simulink model "Single_FLL"  (R2021a)
settings: Solver=VariableStepAuto  StartTime=0.0  StopTime=2  RelTol=1e-3
libraries: dspswit3 x2, spspowerguiLib x1
settings Model: Creator=Swaran Pratap Singh  LastModifiedBy=Swaran Pratap Singh
settings DataIOCC: InspectSignalLogs=on  ReturnWorkspaceOutputs=off

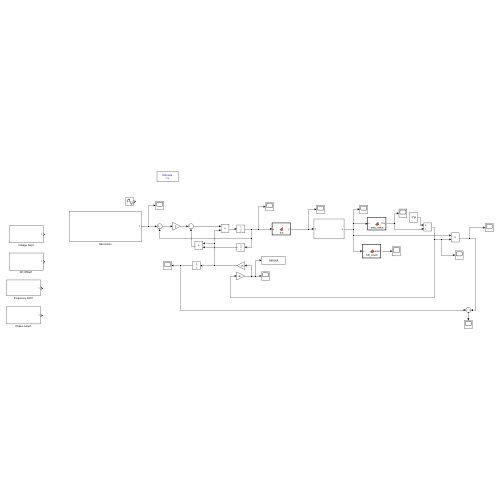
[thumbnail: Simulink's stored preview of the top-level diagram]
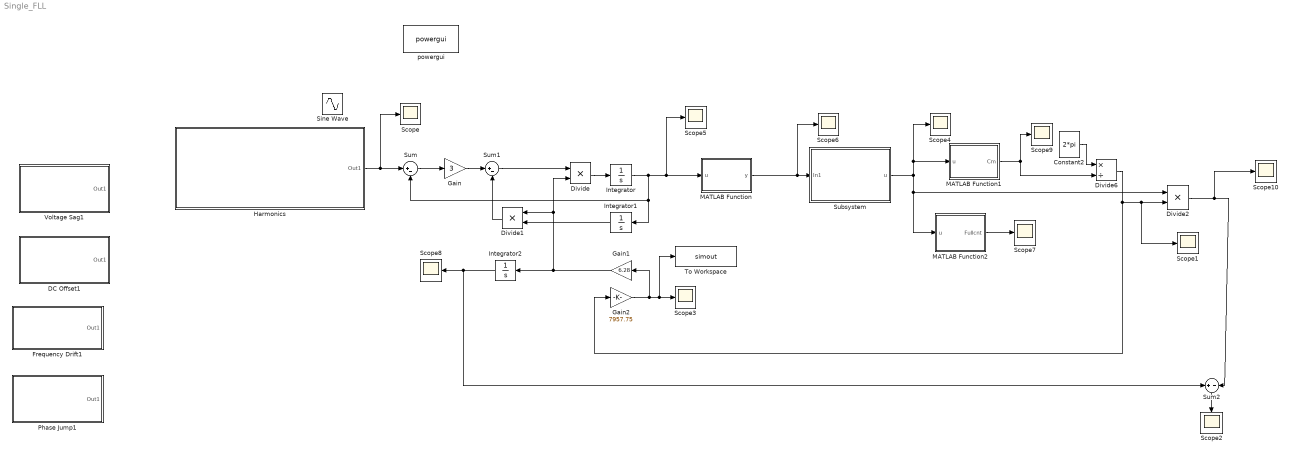
== system Single_FLL ==
  Constant2 : Constant  Value=2*pi
  DC Offset1 : Subsystem
  Divide : Product  Inputs=**
  Divide1 : Product  Inputs=**
  Divide2 : Product  Inputs=**
  Divide6 : Product  Inputs=*/
  Frequency Drift1 : Subsystem
  Gain : Gain  Gain=3
  Gain1 : Gain  Gain=6.28
  Gain2 : Gain  Gain=7957.75
  Harmonics : Subsystem
  Integrator : Integrator
  Integrator1 : Integrator
  Integrator2 : Integrator
  MATLAB Function : MATLAB Function  TreatAsAtomicUnit=on
  MATLAB Function1 : MATLAB Function  TreatAsAtomicUnit=on
  MATLAB Function2 : MATLAB Function  TreatAsAtomicUnit=on
  Phase Jump1 : Subsystem
  Scope{,1..10} (11 alike) : Scope
  Sine Wave : Sin  Amplitude=230  Frequency=2*pi*50  SampleTime=0.000001
  Subsystem : Subsystem
  Sum : Sum  Inputs=|+-
  Sum1 : Sum  Inputs=|+-
  Sum2 : Sum  Inputs=+-
  To Workspace : ToWorkspace  VariableName=simout  SaveFormat=Timeseries  SampleTime=-1
  Voltage Sag1 : Subsystem
  powergui : spspowerguiLib/powergui  Priority=1  SimulationMode=Discrete  SampleTime=1  frequency=60  Iterations=50  frequencyindice=50  Pbase=100e6  ErrMax=1e-4  UnitsV=kV  UnitsW=MW  buscounter=0  FunctionMessages=off  echomessages=off  EnableUseOfTLC=off  CurrentSourceSwitches=off  DisableSnubberDevices=off  DisableRonSwitches=off  DisableVfSwitches=off  DisplayEquations=off  AutomaticDiscreteSolvers=off  SolverType=Tustin/Backward Euler (TBE)  Interpol=off  ExternalGateDelay=off  methode=off  Ts=100  x0status=blocks  SPID=on  SwTol=0  HookPort=off  NonlinearTolerance=1e-4  nMaxIteration=100  ContinueOnMaxIteration=off  RestoreLinks=warning  ResistiveCurrentMeasurement=off  Frange=[0:2:500]  Ylog=off  Xlog=on  ShowGrid=off  save=off  variable=ZData  structure=0  ZoomFFT=off  StartTime=0.0  cycles=1  DisplayStyle=1  fundamental=60  FreqAxis=off  MaxFrequency=1000  frequencyindicesteady=1  RmsSteady=1  display=off
  wires:
  MATLAB Function/1(y) -> Scope6/1, Subsystem/1(In1)
  Subsystem/1(u) -> MATLAB Function1/1(u), Scope4/1, MATLAB Function2/1(u), Divide2/1
  Gain1/1 -> Integrator2/1, Divide1/1, Divide/2
  Sum/1 -> Gain/1
  Divide2/1 -> Scope10/1, Sum2/2
  Integrator1/1 -> Divide1/2
  Divide1/1 -> Sum1/2
  Gain/1 -> Sum1/1
  Constant2/1 -> Divide6/1
  MATLAB Function2/1(Fullcnt) -> Scope7/1
  Divide/1 -> Integrator/1
  Integrator2/1 -> Sum2/1, Scope8/1
  MATLAB Function1/1(Cm) -> Divide6/2, Scope9/1
  Gain2/1 -> To Workspace/1, Scope3/1, Gain1/1
  Sum2/1 -> Scope2/1
  Divide6/1 -> Gain2/1, Scope1/1, Divide2/2
  Sum1/1 -> Divide/1
  Integrator/1 -> Integrator1/1, Sum/2, Scope5/1, MATLAB Function/1(u)
  Harmonics/1(Out1) -> Scope/1, Sum/1

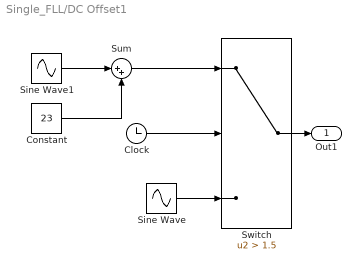
== system Single_FLL/DC Offset1 ==
  Clock : Clock
  Constant : Constant  Value=23
  Sine Wave : Sin  Amplitude=230  Frequency=314.16  SampleTime=0.000001
  Sine Wave1 : Sin  Amplitude=230  Frequency=314.16  SampleTime=0.000001
  Sum : Sum  Inputs=|++
  Switch : Switch  Criteria=u2 > Threshold  Threshold=1.5
  Out1 : Outport
  wires:
  Clock/1 -> Switch/2
  Sine Wave/1 -> Switch/3
  Switch/1 -> Out1/1
  Sine Wave1/1 -> Sum/1
  Constant/1 -> Sum/2
  Sum/1 -> Switch/1

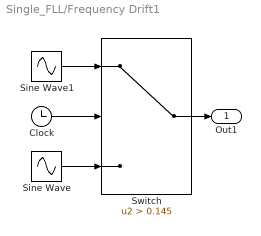
== system Single_FLL/Frequency Drift1 ==
  Clock : Clock
  Sine Wave : Sin  Amplitude=230  Frequency=314.16  SampleTime=0.000001
  Sine Wave1 : Sin  Amplitude=230  Frequency=333.01  Phase=pi  SampleTime=0.000001
  Switch : Switch  Criteria=u2 > Threshold  Threshold=0.145
  Out1 : Outport
  wires:
  Sine Wave1/1 -> Switch/1
  Sine Wave/1 -> Switch/3
  Clock/1 -> Switch/2
  Switch/1 -> Out1/1

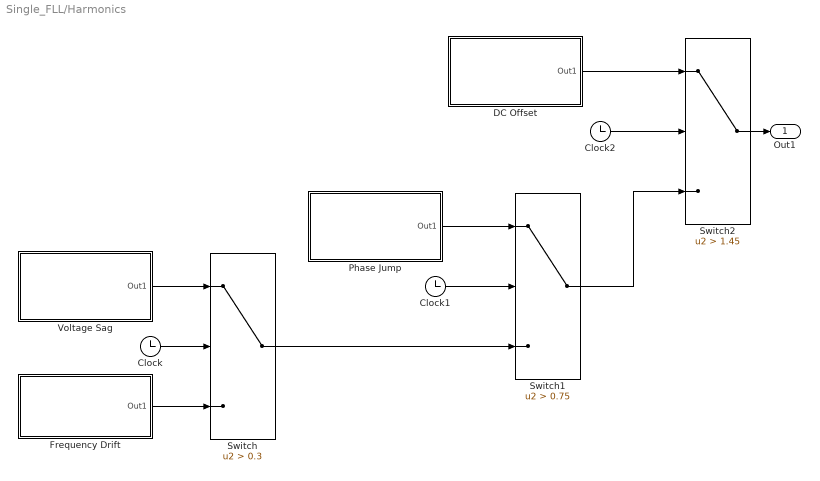
== system Single_FLL/Harmonics ==
  Clock : Clock
  Clock1 : Clock
  Clock2 : Clock
  DC Offset : Subsystem
  Frequency Drift : Subsystem
  Phase Jump : Subsystem
  Switch : Switch  Criteria=u2 > Threshold  Threshold=0.3
  Switch1 : Switch  Criteria=u2 > Threshold  Threshold=0.75
  Switch2 : Switch  Criteria=u2 > Threshold  Threshold=1.45
  Voltage Sag : Subsystem
  Out1 : Outport
  wires:
  Phase Jump/1(Out1) -> Switch1/1
  Switch1/1 -> Switch2/3
  DC Offset/1(Out1) -> Switch2/1
  Switch/1 -> Switch1/3
  Clock/1 -> Switch/2
  Clock1/1 -> Switch1/2
  Frequency Drift/1(Out1) -> Switch/3
  Clock2/1 -> Switch2/2
  Voltage Sag/1(Out1) -> Switch/1
  Switch2/1 -> Out1/1

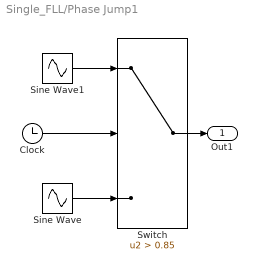
== system Single_FLL/Phase Jump1 ==
  Clock : Clock
  Sine Wave : Sin  Amplitude=230  Frequency=314.16  SampleTime=0.000001
  Sine Wave1 : Sin  Amplitude=230  Frequency=314.16  Phase=0.4167*pi  SampleTime=0.000001
  Switch : Switch  Criteria=u2 > Threshold  Threshold=0.85
  Out1 : Outport
  wires:
  Clock/1 -> Switch/2
  Sine Wave1/1 -> Switch/1
  Sine Wave/1 -> Switch/3
  Switch/1 -> Out1/1

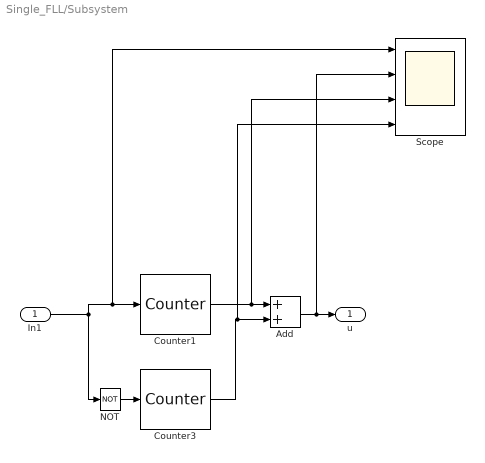
== system Single_FLL/Subsystem ==
  In1 : Inport
  Add : Sum
  Counter1 : dspswit3/Counter  Direction=Up  CountEvent=Free running  CounterSize=User defined  MaxCount=10000  InitialCount=0  Output=Count  HitValue=32  ResetInput=on  SamplesPerFrame=1  Ts=0.00001  CntDtype=double  HitDtype=Logical
  Counter3 : dspswit3/Counter  Direction=Up  CountEvent=Free running  CounterSize=User defined  MaxCount=10000  InitialCount=0  Output=Count  HitValue=32  ResetInput=on  SamplesPerFrame=1  Ts=0.00001  CntDtype=double  HitDtype=Logical
  NOT : Logic  Operator=NOT  IconShape=distinctive  AllPortsSameDT=off  OutDataTypeStr=boolean
  Scope : Scope  NumInputPorts=4
  u : Outport
  wires:
  NOT/1 -> Counter3/1
  Counter3/1 -> Scope/4, Add/2
  Counter1/1 -> Scope/3, Add/1
  In1/1 -> NOT/1, Scope/1, Counter1/1
  Add/1 -> Scope/2, u/1

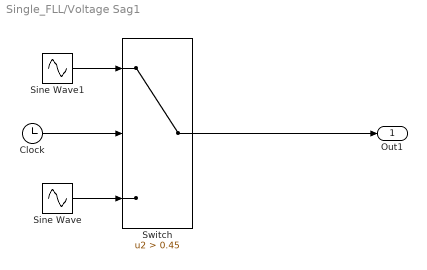
== system Single_FLL/Voltage Sag1 ==
  Clock : Clock
  Sine Wave : Sin  Amplitude=230  Frequency=314.16  SampleTime=0.000001
  Sine Wave1 : Sin  Amplitude=138  Frequency=314.16  SampleTime=0.000001
  Switch : Switch  Criteria=u2 > Threshold  Threshold=0.45
  Out1 : Outport
  wires:
  Clock/1 -> Switch/2
  Sine Wave1/1 -> Switch/1
  Sine Wave/1 -> Switch/3
  Switch/1 -> Out1/1

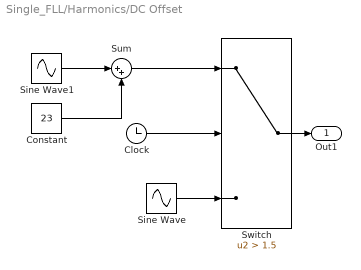
== system Single_FLL/Harmonics/DC Offset ==
  Clock : Clock
  Constant : Constant  Value=23
  Sine Wave : Sin  Amplitude=230  Frequency=314.16  SampleTime=0.000001
  Sine Wave1 : Sin  Amplitude=230  Frequency=314.16  SampleTime=0.000001
  Sum : Sum  Inputs=|++
  Switch : Switch  Criteria=u2 > Threshold  Threshold=1.5
  Out1 : Outport
  wires:
  Clock/1 -> Switch/2
  Sine Wave/1 -> Switch/3
  Switch/1 -> Out1/1
  Sine Wave1/1 -> Sum/1
  Constant/1 -> Sum/2
  Sum/1 -> Switch/1

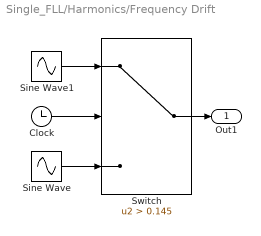
== system Single_FLL/Harmonics/Frequency Drift ==
  Clock : Clock
  Sine Wave : Sin  Amplitude=230  Frequency=314.16  SampleTime=0.000001
  Sine Wave1 : Sin  Amplitude=230  Frequency=333.01  Phase=pi  SampleTime=0.000001
  Switch : Switch  Criteria=u2 > Threshold  Threshold=0.145
  Out1 : Outport
  wires:
  Sine Wave1/1 -> Switch/1
  Sine Wave/1 -> Switch/3
  Clock/1 -> Switch/2
  Switch/1 -> Out1/1

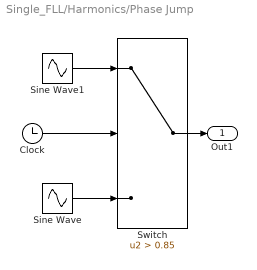
== system Single_FLL/Harmonics/Phase Jump ==
  Clock : Clock
  Sine Wave : Sin  Amplitude=230  Frequency=314.16  SampleTime=0.000001
  Sine Wave1 : Sin  Amplitude=230  Frequency=314.16  Phase=0.4167*pi  SampleTime=0.000001
  Switch : Switch  Criteria=u2 > Threshold  Threshold=0.85
  Out1 : Outport
  wires:
  Clock/1 -> Switch/2
  Sine Wave1/1 -> Switch/1
  Sine Wave/1 -> Switch/3
  Switch/1 -> Out1/1

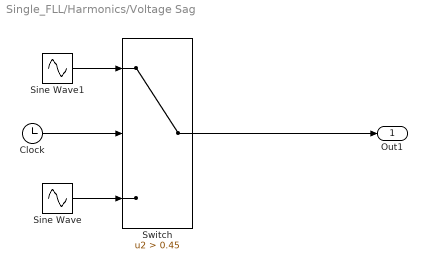
== system Single_FLL/Harmonics/Voltage Sag ==
  Clock : Clock
  Sine Wave : Sin  Amplitude=230  Frequency=314.16  SampleTime=0.000001
  Sine Wave1 : Sin  Amplitude=138  Frequency=314.16  SampleTime=0.000001
  Switch : Switch  Criteria=u2 > Threshold  Threshold=0.45
  Out1 : Outport
  wires:
  Clock/1 -> Switch/2
  Sine Wave1/1 -> Switch/1
  Sine Wave/1 -> Switch/3
  Switch/1 -> Out1/1

== matlab function Single_FLL/MATLAB Function1 ==
  data: u input; Cm output
function Cm = max_value(u)

persistent pre_u
persistent Cm_prev
flag = 1; % Remove int8 and initialization

if isempty(pre_u)
    pre_u = 1;
    Cm_prev=1;
end

if (pre_u > u)
    %Cm = pre_u;
    flag = 0;
else 
    %Cm = u;
    flag = 1;
end
%pre_u = Cm;
if (flag == 0)
    Cm = pre_u;
    Cm_prev=Cm;
    pre_u=u;
    flag = 1;
else
    pre_u=u;
    if(Cm_prev~=1)

        Cm=Cm_prev;
    else 
        Cm=pre_u;
    end
end
   
end

== matlab function Single_FLL/MATLAB Function ==
  data: u input; y output
function y = fcn(u)
    if u > 0
        y = 1;
    else
       y = 0;
    end
end

== matlab function Single_FLL/MATLAB Function2 ==
  data: u input; Fullcnt output
function   Fullcnt = full_count(u)

persistent pre_u
persistent Cm_prev
persistent cnt  
persistent Cm
flag = 1; % Remove int8 and initialization

if isempty(pre_u)
    pre_u = -1;
    Cm_prev=1;
    cnt=0;
    
end

if (pre_u > u)
    %Cm = pre_u;
    flag = 0;
else 
    %Cm = u;
    flag = 1;
end
%pre_u = Cm;
if (flag == 0)
    if(mod(cnt,2)==0)
        Cm = pre_u;
        Cm_prev=Cm;
    else
        Cm=Cm_prev;
    end
    pre_u=u;
    flag = 1;
    cnt=cnt+1;
else
    pre_u=u;
    if(Cm_prev~=1)

        Cm=Cm_prev;
    else 
    
            Cm=pre_u;

    end
end
if(mod(cnt,2)==1)
    Fullcnt=u+Cm;
else
    Fullcnt=u;
end
   
end
